simulink model "test1"  (R2023b)
settings: Solver=VariableStepAuto  StartTime=0.0  StopTime=100000  RelTol=1e-3
values from neighbouring files (symbols this model uses):
  bhi = fir2(59,f,mhi)    [gen_fir.m]
  cnt1_max = 63    [TEST1_INIT.m]
libraries: hdlsllib x2, dsphdlfiltering2 x1
settings Model: Creator=31651  LastModifiedBy=31651
settings OptimizationCC: BlockReduction=off  ConditionallyExecuteInputs=off  DefaultParameterBehavior=Inlined
settings DebuggingCC: AlgebraicLoopMsg=error
settings HardwareCC: ProdBitPerPointer=32  ProdBitPerSizeT=32  ProdBitPerPtrDiffT=32  ProdLargestAtomicFloat=None  ProdIntDivRoundTo=Undefined  ProdEndianess=Unspecified  ProdWordSize=32  ProdHWDeviceType=ASIC/FPGA->ASIC/FPGA  TargetBitPerPointer=64  TargetBitPerSizeT=64  TargetBitPerPtrDiffT=64  TargetLongLongMode=on  TargetIntDivRoundTo=Zero  TargetEndianess=LittleEndian  TargetWordSize=64  TargetHWDeviceType=Custom Processor->MATLAB Host Computer  ProdEqTarget=off

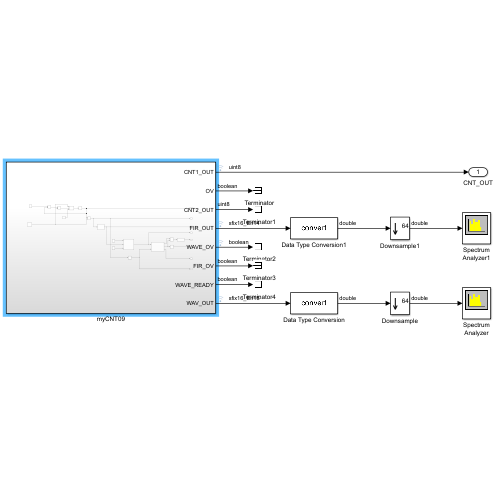
[thumbnail: Simulink's stored preview of the top-level diagram]
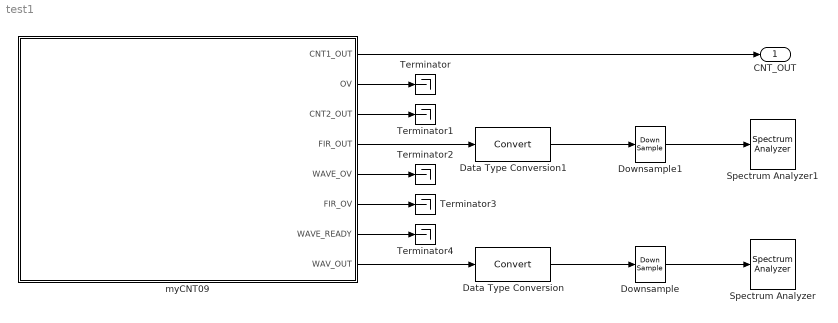
== system test1 ==
  Data Type Conversion : DataTypeConversion  SaturateOnIntegerOverflow=off  RndMeth=Floor  LockScale=on
  Data Type Conversion1 : DataTypeConversion  SaturateOnIntegerOverflow=off  RndMeth=Floor  LockScale=on
  Downsample : DownSample  N=64  RateOptions=Allow multirate processing
  Downsample1 : DownSample  N=64  RateOptions=Allow multirate processing
  Spectrum Analyzer : SpectrumAnalyzer  WindowPosition=[368.000000,182.000000,800.000000,500.000000,]  ScopeFrameLocation=window  Span=0.03125  StartFrequency=-0.015625  StopFrequency=0.015625  YLimits=[-3603.44492261,-2802.67938425]
  Spectrum Analyzer1 : SpectrumAnalyzer  WindowPosition=[235.000000,112.000000,800.000000,500.000000,]  ScopeFrameLocation=window  Span=0.016666666666666666  StartFrequency=-0.008333333333333333  StopFrequency=0.008333333333333333  YLimits=[-3603.44492261,-2802.67938425]
  Terminator{,1..4} (5 alike) : Terminator
  myCNT09 : Subsystem
  CNT_OUT : Outport  VectorParamsAs1DForOutWhenUnconnected=off
  wires:
  myCNT09/1(CNT1_OUT) -> CNT_OUT/1
  myCNT09/3(CNT2_OUT) -> Terminator1/1
  myCNT09/2(OV) -> Terminator/1
  myCNT09/5(WAVE_OV) -> Terminator2/1
  Downsample/1 -> Spectrum Analyzer/1
  Data Type Conversion/1 -> Downsample/1
  myCNT09/8(WAV_OUT) -> Data Type Conversion/1
  myCNT09/7(WAVE_READY) -> Terminator4/1
  myCNT09/6(FIR_OV) -> Terminator3/1
  myCNT09/4(FIR_OUT) -> Data Type Conversion1/1
  Data Type Conversion1/1 -> Downsample1/1
  Downsample1/1 -> Spectrum Analyzer1/1

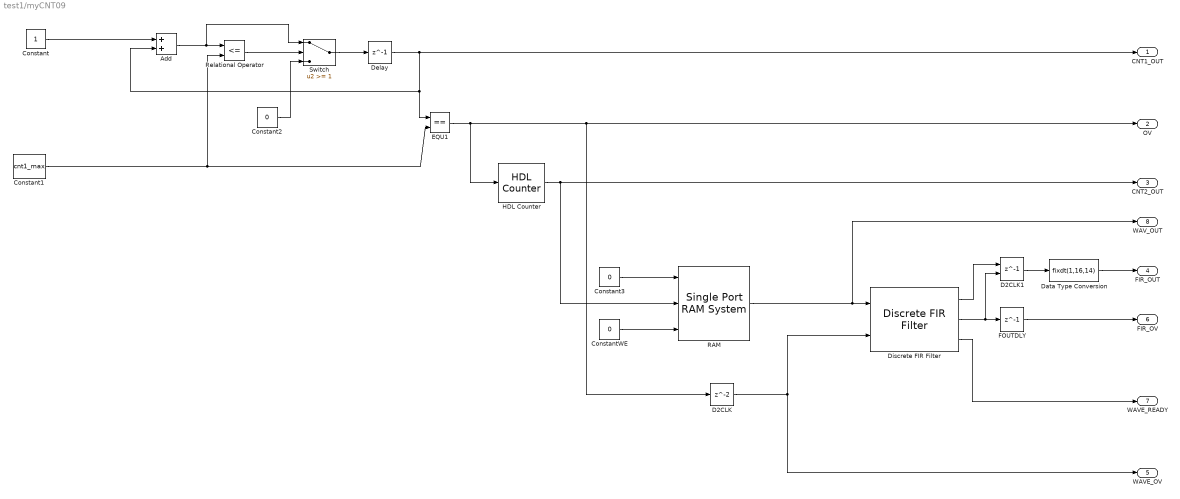
== system test1/myCNT09 ==
  Add : Sum  OutDataTypeStr=uint8
  Constant : Constant  OutDataTypeStr=uint8  SampleTime=1
  Constant1 : Constant  Value=cnt1_max  OutDataTypeStr=uint8  SampleTime=1
  Constant2 : Constant  Value=0  OutDataTypeStr=uint8  SampleTime=1
  Constant3 : Constant  Value=0  OutDataTypeStr=fixdt(1,16,15)  SampleTime=1
  ConstantWE : Constant  Value=0  OutDataTypeStr=boolean  SampleTime=1
  D2CLK : Delay  InitialCondition=0
  D2CLK1 : Delay  DelayLength=1  InitialCondition=0  ShowEnablePort=on
      settings: InputPortMap=u0,e6
  Data Type Conversion : DataTypeConversion  OutDataTypeStr=fixdt(1,16,14)  SaturateOnIntegerOverflow=off  RndMeth=Floor
  Delay : Delay  DelayLength=1  InitialCondition=0
  Discrete FIR Filter : dsphdlfiltering2/Discrete FIR Filter  NumeratorSource=Property  Numerator=bhi  NumeratorPrototype=[]  FilterStructure=Partly serial systolic  SerializationOption=Maximum number of multipliers  NumCycles=2  NumberOfMultipliers=3  SimulateUsing=Code generation  roundingMode=Floor  overflowMode=off  CoefficientsDataTypeStr=Inherit: Same word length as input  OutputDataTypeStr=Inherit: Same word length as input  ResetInputPort=off  HDLGlobalReset=off  CoeffMultiplier=Multiplier  UseMultForPow2Coeff=on
  EQU1 : RelationalOperator  Operator===  InputSameDT=off
  FOUTDLY : Delay  DelayLength=1  InitialCondition=0
  HDL Counter : hdlsllib/Sources/HDL Counter  CountType=Count limited  CountInit=0  CountStep=1  CountMax=cnt2_max  CountFromType=Initial value  CountFrom=0  CountResetPort=off  CountLoadPort=off  CountEnbPort=on  CountDirPort=off  CountHitOutputPort=off  CountDataType=Unsigned  CountWordLen=8  CountFracLen=0  CountSampTime=1
  RAM : hdlsllib/HDL RAMs/Single Port RAM System  RAMType=Single port  AsyncRead=off  WriteOutputValue=New data  RAMInitialValue=vec_1  allowBusInputs=off  WritesHaveOutput=on  NumReads=0  NumWrites=1  SimulateUsing=Code generation
  Relational Operator : RelationalOperator  Operator=<=  OutDataTypeStr=boolean  InputSameDT=off
  Switch : Switch  Threshold=1  OutDataTypeStr=uint8  SaturateOnIntegerOverflow=off  InputSameDT=off
  CNT1_OUT : Outport  OutDataTypeStr=uint8  VectorParamsAs1DForOutWhenUnconnected=off
  OV : Outport  Port=2  VectorParamsAs1DForOutWhenUnconnected=off
  CNT2_OUT : Outport  Port=3
  FIR_OUT : Outport  Port=4  VectorParamsAs1DForOutWhenUnconnected=off
  WAVE_OV : Outport  Port=5  VectorParamsAs1DForOutWhenUnconnected=off
  FIR_OV : Outport  Port=6  VectorParamsAs1DForOutWhenUnconnected=off
  WAVE_READY : Outport  Port=7  VectorParamsAs1DForOutWhenUnconnected=off
  WAV_OUT : Outport  Port=8
  wires:
  Switch/1 -> Delay/1
  Relational Operator/1 -> Switch/2
  Add/1 -> Switch/1, Relational Operator/1
  Delay/1 -> EQU1/1, Add/2, CNT1_OUT/1
  Constant/1 -> Add/1
  Constant1/1 -> EQU1/2, Relational Operator/2
  Constant2/1 -> Switch/3
  EQU1/1 -> HDL Counter/1, D2CLK/1, OV/1
  HDL Counter/1 -> RAM/2, CNT2_OUT/1
  ConstantWE/1 -> RAM/3
  Constant3/1 -> RAM/1
  Discrete FIR Filter/1 -> D2CLK1/1
  D2CLK/1 -> Discrete FIR Filter/2, WAVE_OV/1
  Discrete FIR Filter/2 -> FOUTDLY/1, D2CLK1/2
  Discrete FIR Filter/3 -> WAVE_READY/1
  D2CLK1/1 -> Data Type Conversion/1
  FOUTDLY/1 -> FIR_OV/1
  RAM/1 -> WAV_OUT/1, Discrete FIR Filter/1
  Data Type Conversion/1 -> FIR_OUT/1
